simulink library "Hot_Water_T_Mdot_Profile"  (R2018b)
settings: Solver=ode45  StartTime=0.0  StopTime=10.0  RelTol=1e-3  EnableMultiTasking=on
libraries: carnot x5
settings Model: Creator=lena.frank  LastModifiedBy=P41573
settings DataIOCC: LimitDataPoints=on  SaveFormat=Array  SignalLoggingSaveFormat=ModelDataLogs
settings OptimizationCC: ExpressionDepthLimit=2147483647  LifeSpan=inf
settings DebuggingCC: UnderspecifiedInitializationDetection=Classic  MergeDetectMultiDrivingBlocksExec=none  SolverPrmCheckMsg=warning  FcnCallInpInsideContextMsg=warning  StateNameClashWarn=warning  SFUnexpectedBacktrackingDiag=warning  SFNoUnconditionalDefaultTransitionDiag=warning  SFExecutionAtInitializationDiag=none
settings HardwareCC: ProdBitPerPointer=32  ProdBitPerSizeT=32  ProdBitPerPtrDiffT=32  ProdLargestAtomicFloat=None  ProdIntDivRoundTo=Undefined  ProdEndianess=Unspecified  ProdWordSize=32  ProdHWDeviceType=32-bit Generic
settings ModelReferenceCC: PropagateSignalLabelsOutOfModel=off
settings SFSimCC: SimUseLocalCustomCode=off
settings RTWCC: RTWUseLocalCustomCode=off
settings CodeAppCC: StateflowObjectComments=on
settings GRTTargetCC: TargetLangStandard=C89/C90 (ANSI)  GeneratePreprocessorConditionals=Disable all  CombineOutputUpdateFcns=off  GRTInterface=on
settings ConfigComp: CovMetricSettings=dw  CovHtmlReporting=on  CovSaveCumulativeToWorkspaceVar=on  CovSaveSingleToWorkspaceVar=on  CovExternalEMLEnable=off

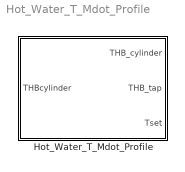
== system Hot_Water_T_Mdot_Profile ==
  Hot_Water_T_Mdot_Profile : Subsystem  VariantControl=Variant3  mask(Hot Water T-Mdot Profile){Thot=45, Tcold=10, Tamp=0, dshift=0, period=24*3600   % one day, rep_seq_t=0  % tapping at 0:00, rep_seq_d=1*3600  % total duration is 2 h, rep_seq_y=1*10/60   % 10 kg/min}
      mask prompts: Thot "Tapping temperature setpoint in °C"; Tcold "Mean temperature in °C"; Tamp "Amplitude of the sine in K"; dshift "Phase shift of the sine in [days]"; period "Period of the sequence in s"; rep_seq_t "Time values tapping start in s"; rep_seq_d "Duration of each tapping in s"; rep_seq_y "Massflow of each tapping in kg/s"
      mask help:
      | Hot water consumption with a temperature and massflow profile.
      | The hot water of the cylinder entering the block is mixed with the cold water to reach the temperature setpoint. The necessary massflow through the cylinder is calculated by this block and set in the outport to the cylinder.
      mask TypeOptions Thot: T_hot_water/Value
      mask TypeOptions Tcold: T_cold_Water_Sine/T
      mask TypeOptions Tamp: T_cold_Water_Sine/Tamp
      mask TypeOptions dshift: T_cold_Water_Sine/dshift
      mask TypeOptions period: mdot_rep_seq/period
      mask TypeOptions rep_seq_t: mdot_rep_seq/rep_seq_t
      mask TypeOptions rep_seq_d: mdot_rep_seq/rep_seq_d
      mask TypeOptions rep_seq_y: mdot_rep_seq/rep_seq_y
      mask DialogControl Container3 Prompt: Cold water parameters
      mask DialogControl Container4 Prompt: Repeating sequence for masslfow
      mask Display:
      | text(15,120,'T-Mdot-Profile')
      | plot(0,0,140,130,[70,76,78,63,65,70,70,10],[80,78,74,74,78,80,100,100],[23,23,20,10],[43,47,50,50],[10,10,20,28,30,10],[30,20,20,23,30,30],[22,17],[54,54],[20,20],[54,50],[90,90,50,50],[10,-0,-0,10],[63,64],[60,72],[61,62],[38,50],[60,61],[13,27],[90,85,81,76,70,65,59,54,50],[6,4,6,4,6,4,5,3,5],[68,69],[56,68],[68,68],[32,44],[67,67],[13,23],[73,73],[61,71],[73,73],[43,52],[74,73],[21,36],[78,77],[56,67],[79,79],[34,45],[78,77],[9,23],[82,81],[14,26])

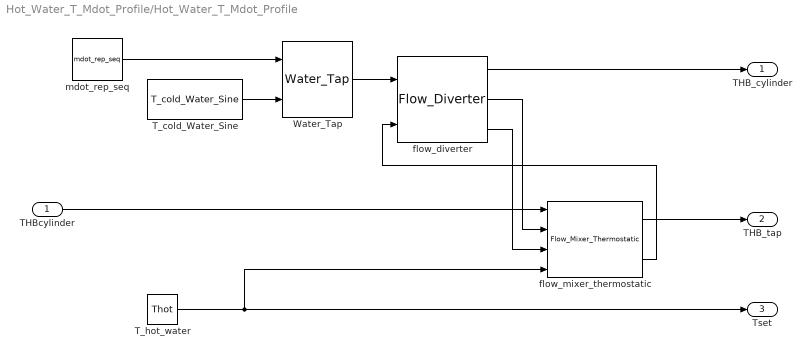
== system Hot_Water_T_Mdot_Profile/Hot_Water_T_Mdot_Profile ==
  THBcylinder : Inport
  T_cold_Water_Sine : carnot/Load/Hot_Water_Tapping/T_cold_Water_Sine  T=Tcold  Tamp=Tamp  dshift=dshift
      settings: SourceProductName=Carnot
  T_hot_water : Constant  Value=Thot
  Water_Tap : carnot/Load/Hot_Water_Tapping/Water_Tap  dia=0.02  p=2e5
      settings: SourceProductName=Carnot
  flow_diverter : carnot/Hydraulics/Flow_Diverter
      settings: SourceProductName=Carnot
  flow_mixer_thermostatic : carnot/Hydraulics/Flow_Mixer_Thermostatic  t=10
      settings: SourceProductName=Carnot
  mdot_rep_seq : carnot/Load/Hot_Water_Tapping/mdot_rep_seq  period=period  rep_seq_t=rep_seq_t  rep_seq_d=rep_seq_d  rep_seq_y=rep_seq_y
      settings: SourceProductName=Carnot
  THB_cylinder : Outport
  THB_tap : Outport  Port=2
  Tset : Outport  Port=3
  wires:
  mdot_rep_seq/1 -> Water_Tap/1
  T_cold_Water_Sine/1 -> Water_Tap/2
  T_hot_water/1 -> Tset/1, flow_mixer_thermostatic/4
  Water_Tap/1 -> flow_diverter/1
  flow_mixer_thermostatic/2 -> flow_diverter/2
  flow_mixer_thermostatic/1 -> THB_tap/1
  THBcylinder/1 -> flow_mixer_thermostatic/1
  flow_diverter/1 -> THB_cylinder/1
  flow_diverter/2 -> flow_mixer_thermostatic/2
  flow_diverter/3 -> flow_mixer_thermostatic/3
